simulink model "StereoImageRectificationHDL2020a"  (R2020a)
settings: Solver=FixedStepDiscrete  StartTime=0.0  StopTime=totalPixels*totalLines  FixedStep=1  RelTol=1e-3
InitFcn:
  | load('stereoParams.mat');
  | img = imread(get_param('StereoImageRectificationHDL2020a/LeftInputImage','FileName'));
  | dimOut=size(img);
  | [imgRowSize, imgColSize] = size(img);
  | run('ComputeRectificationParams.m');
values from neighbouring files (symbols this model uses):
  displacement = maxDev+firstRow    [ComputeRectificationParams.m]
  distCoeffsL = [this.CameraParameters1.RadialDistortion, this.CameraParameters1.TangentialDistortion]    [ComputeRectificationParams.m]
  distCoeffsR = [this.CameraParameters2.RadialDistortion, this.CameraParameters2.TangentialDistortion]    [ComputeRectificationParams.m]
  offset = displacement+50    [ComputeRectificationParams.m]
  recleftfx = 1/intrinsicL(1,1)    [ComputeRectificationParams.m]
  recleftfy = 1/intrinsicL(2,2)    [ComputeRectificationParams.m]
  recrightfx = 1/intrinsicR(1,1)    [ComputeRectificationParams.m]
  recrightfy = 1/intrinsicR(2,2)    [ComputeRectificationParams.m]
  totalLines = R + 100    (= 580)    [setup.m]
  totalPixels = C + frontPorch    (= 802)    [setup.m]
undefined symbols (not defined in the file or in its folder): gray, imgColSize, imgRowSize, intrinsicL, intrinsicR, leftH, rightH, XBounds, YBounds
libraries: simulink x62, hdlsllib x30, visionhdlio x4, visionsources x2, visionhdlutilities x1
(part 2 of 3)

== system StereoImageRectificationHDL2020a/HDLStereoImageRectification/RightUndistortion/Normalization ==
  yCoordinate : Inport
  xCoordinate : Inport  Port=2
  Add : Sum  Inputs=+-
  Add1 : Sum  Inputs=+-
  Constant : Constant  Value=intrinsic(2,3)  OutDataTypeStr=fixdt(1,ceil(log2(intrinsic(2,3)))+24,23)  SampleTime=-1
  Constant1 : Constant  Value=intrinsic(1,3)  OutDataTypeStr=fixdt(1,ceil(log2(intrinsic(1,3)))+24,23)  SampleTime=-1
  Constant2 : Constant  Value=recfy  OutDataTypeStr=Inherit: Inherit via back propagation  SampleTime=-1
  Constant3 : Constant  Value=recfx  OutDataTypeStr=Inherit: Inherit via back propagation  SampleTime=-1
  Delay{1..3,8} (4 alike) : Delay
  Delay30 : Delay  DelayLength=1
  Delay31 : Delay  DelayLength=1
  Product13 : Product  OutDataTypeStr=Inherit: Same as first input
  Product14 : Product  OutDataTypeStr=Inherit: Same as first input
  yNorm : Outport
  xNorm : Outport  Port=2
  wires:
  Delay2/1 -> xNorm/1
  Delay1/1 -> yNorm/1
  xCoordinate/1 -> Delay31/1
  Product14/1 -> Delay2/1  "xNorm"
  Add/1 -> Delay8/1
  Product13/1 -> Delay1/1  "yNorm"
  Delay30/1 -> Add/1
  Delay31/1 -> Add1/1
  Delay8/1 -> Product13/1
  yCoordinate/1 -> Delay30/1
  Constant2/1 -> Product13/2
  Constant3/1 -> Product14/2
  Constant/1 -> Add/2
  Add1/1 -> Delay3/1
  Delay3/1 -> Product14/1
  Constant1/1 -> Add1/2

== system StereoImageRectificationHDL2020a/HDLStereoImageRectification/RightUndistortion/ParameterCalculation ==
  yNorm : Inport
  xNorm : Inport  Port=2
  Add2 : Sum
  Delay{1..4,6..7,9} (7 alike) : Delay
  Product{,10..12} (4 alike) : Product  OutDataTypeStr=Inherit: Inherit via back propagation
  r4 : Outport
  r2 : Outport  Port=2
  xyProduct : Outport  Port=3
  xNorm2 : Outport  Port=4
  yNorm2 : Outport  Port=5
  wires:
  Delay4/1 -> xNorm2/1
  Delay3/1 -> yNorm2/1
  Delay2/1 -> xyProduct/1
  Delay1/1 -> Delay2/1
  xNorm/1 -> Product/2, Product11/1, Product11/2
  Product/1 -> Delay1/1  "xyProduct"
  yNorm/1 -> Product/1, Product10/2, Product10/1
  Add2/1 -> Delay9/1  "r2"
  Delay6/1 -> Delay3/1, Add2/1
  Delay7/1 -> Add2/2, Delay4/1
  Delay9/1 -> Product12/2, r2/1, Product12/1
  Product12/1 -> r4/1  "r4"
  Product11/1 -> Delay7/1  "xNorm2"
  Product10/1 -> Delay6/1  "yNorm2"

== system StereoImageRectificationHDL2020a/HDLStereoImageRectification/RightUndistortion/RadialDistortion ==
  r4 : Inport
  r2 : Inport  Port=2
  Add3 : Sum
  Delay{10..13,18} (5 alike) : Delay
  Product1 : Product  OutDataTypeStr=Inherit: Same as first input
  Product2 : Product  OutDataTypeStr=Inherit: Same as first input
  radial1 : Constant  Value=distCoeffs(1)  OutDataTypeStr=fixdt(1,17,16)  SampleTime=-1
  radial2 : Constant  Value=distCoeffs(2)  OutDataTypeStr=fixdt(1,17,16)  SampleTime=-1
  alpha : Outport
  wires:
  Delay10/1 -> Product1/1
  Delay12/1 -> Add3/1
  radial1/1 -> Product1/2
  Delay18/1 -> alpha/1
  Delay11/1 -> Product2/1
  Product2/1 -> Delay12/1
  r4/1 -> Delay11/1
  radial2/1 -> Product2/2
  Delay13/1 -> Add3/2
  Product1/1 -> Delay13/1
  Add3/1 -> Delay18/1  "alpha"
  r2/1 -> Delay10/1

== system StereoImageRectificationHDL2020a/HDLStereoImageRectification/RightUndistortion/dxTangential ==
  r2 : Inport
  xyProd : Inport  Port=2
  xNorm2 : Inport  Port=3
  Add : Sum
  Add1 : Sum
  Delay{,1..4,6..7} (7 alike) : Delay
  Delay5 : Delay  DelayLength=1
  Product : Product  OutDataTypeStr=Inherit: Same as first input
  Product2 : Product  OutDataTypeStr=Inherit: Same as first input  LockScale=on
  Shift Arithmetic : ArithShift  BitShiftNumber=1  BitShiftDirection=Left
  Shift Arithmetic1 : ArithShift  BitShiftNumber=1  BitShiftDirection=Left
  tangential1 : Constant  Value=distCoeffs(3)  OutDataTypeStr=fixdt(1,17,15)  SampleTime=-1
  tangential2 : Constant  Value=distCoeffs(4)  OutDataTypeStr=fixdt(1,17,15)  SampleTime=-1
  dxTan : Outport
  wires:
  Delay7/1 -> Delay3/1
  Delay6/1 -> Shift Arithmetic1/1
  tangential1/1 -> Product/2
  Shift Arithmetic1/1 -> Delay7/1
  Delay5/1 -> dxTan/1
  Add1/1 -> Delay5/1
  Delay4/1 -> Add1/2
  Product2/1 -> Delay4/1
  Delay3/1 -> Add1/1
  Product/1 -> Delay6/1
  tangential2/1 -> Product2/2
  Delay2/1 -> Product2/1
  Add/1 -> Delay2/1
  Delay1/1 -> Add/2
  r2/1 -> Delay1/1
  Delay/1 -> Add/1
  Shift Arithmetic/1 -> Delay/1
  xNorm2/1 -> Shift Arithmetic/1
  xyProd/1 -> Product/1

== system StereoImageRectificationHDL2020a/HDLStereoImageRectification/RightUndistortion/dyTangential ==
  r2 : Inport
  xyProd : Inport  Port=2
  yNorm2 : Inport  Port=3
  Add : Sum
  Add1 : Sum
  Delay{,1..4,6..7} (7 alike) : Delay
  Delay5 : Delay  DelayLength=1
  Product : Product  OutDataTypeStr=Inherit: Same as first input
  Product2 : Product  OutDataTypeStr=Inherit: Same as first input
  Shift Arithmetic : ArithShift  BitShiftNumber=1  BitShiftDirection=Left
  Shift Arithmetic1 : ArithShift  BitShiftNumber=1  BitShiftDirection=Left
  tangential1 : Constant  Value=distCoeffs(3)  OutDataTypeStr=fixdt(1,17,15)  SampleTime=-1
  tangential2 : Constant  Value=distCoeffs(4)  OutDataTypeStr=fixdt(1,17,15)  SampleTime=-1
  dyTan : Outport
  wires:
  Delay7/1 -> Delay3/1
  Delay6/1 -> Shift Arithmetic1/1
  Product/1 -> Delay6/1
  Shift Arithmetic1/1 -> Delay7/1
  Delay5/1 -> dyTan/1
  Add1/1 -> Delay5/1
  Delay4/1 -> Add1/2
  Product2/1 -> Delay4/1
  Delay3/1 -> Add1/1
  tangential1/1 -> Product2/2
  Delay2/1 -> Product2/1
  Add/1 -> Delay2/1
  Delay1/1 -> Add/2
  r2/1 -> Delay1/1
  Delay/1 -> Add/1
  Shift Arithmetic/1 -> Delay/1
  yNorm2/1 -> Shift Arithmetic/1
  tangential2/1 -> Product/2
  xyProd/1 -> Product/1

== system StereoImageRectificationHDL2020a/HDLStereoImageRectification/LeftInterpolation/AddressGeneration/AddressCalculation ==
  col : Inport
  row : Inport  Port=2
  Add4 : Sum  OutDataTypeStr=Inherit: Same as first input
  CappingAddress : Subsystem
  Constant2 : Constant  OutDataTypeStr=Inherit: Inherit via back propagation  SampleTime=-1
  Delay{,1..3} (4 alike) : Delay  DelayLength=3
  IndexChangeForMemoryAccess : MATLAB Function  TreatAsAtomicUnit=on
  Pix1Add : Subsystem
  Pix2Add : Subsystem
  Pix3Add : Subsystem
  Pix4Add : Subsystem
  Vector Concatenate : Concatenate  NumInputs=4
  Vector Concatenate1 : Concatenate  NumInputs=4
  leftAdd : Outport
  leftIndex : Outport  Port=2
  wires:
  Constant2/1 -> Add4/2
  IndexChangeForMemoryAccess/1(Add_Re) -> leftAdd/1
  Vector Concatenate/1 -> IndexChangeForMemoryAccess/1(add)
  Vector Concatenate1/1 -> IndexChangeForMemoryAccess/2(index)
  row/1 -> CappingAddress/1(row)
  col/1 -> CappingAddress/2(col)
  CappingAddress/1(r) -> Add4/1, Pix1Add/1(row)
  CappingAddress/2(c) -> Pix3Add/2(col), Pix1Add/2(col)
  IndexChangeForMemoryAccess/2(Index_Re) -> leftIndex/1
  Pix1Add/1(A1) -> Pix2Add/1(A1), Delay/1
  Pix1Add/2(index) -> Pix2Add/2(Index), Delay2/1
  Add4/1 -> Pix3Add/1(row)
  Pix3Add/1(A3) -> Pix4Add/1(A3), Delay1/1
  Pix3Add/2(index) -> Pix4Add/2(Index), Delay3/1
  Pix2Add/1(A2) -> Vector Concatenate/2
  Pix2Add/2(index) -> Vector Concatenate1/2
  Pix4Add/2(index) -> Vector Concatenate1/4
  Pix4Add/1(A4) -> Vector Concatenate/4
  Delay/1 -> Vector Concatenate/1
  Delay1/1 -> Vector Concatenate/3
  Delay2/1 -> Vector Concatenate1/1
  Delay3/1 -> Vector Concatenate1/3

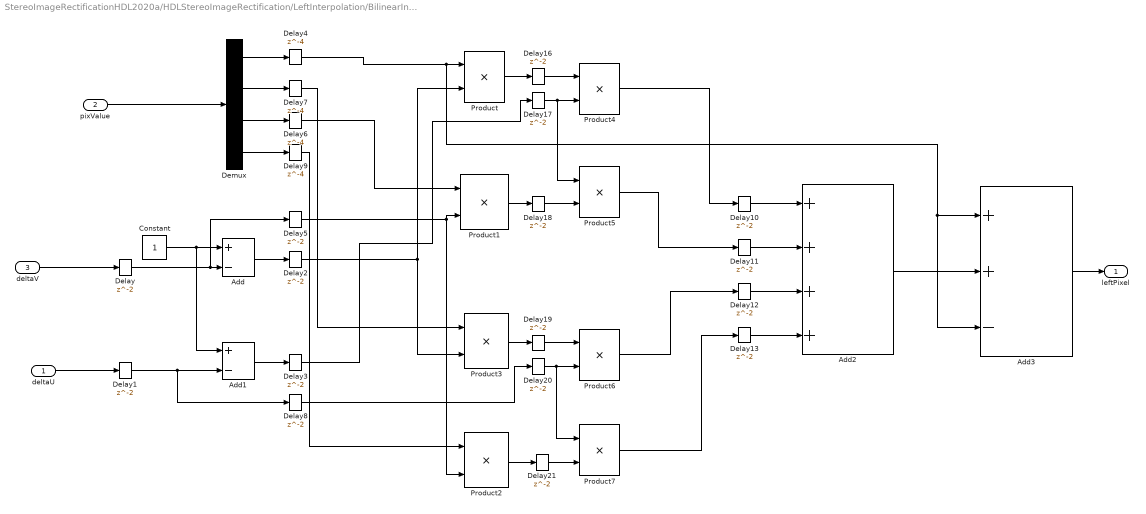
== system StereoImageRectificationHDL2020a/HDLStereoImageRectification/LeftInterpolation/BilinearInterpolation/BilinearInterpolationEquation ==
  deltaU : Inport
  pixValue : Inport  Port=2
  deltaV : Inport  Port=3
  Add : Sum  Inputs=+-  OutDataTypeStr=Inherit: Inherit via back propagation
  Add1 : Sum  Inputs=+-  OutDataTypeStr=Inherit: Inherit via back propagation
  Add2 : Sum  Inputs=++++  OutDataTypeStr=Inherit: Inherit via back propagation  RndMeth=Nearest
  Add3 : Sum  Inputs=++-  RndMeth=Nearest  OutDataTypeStr=Inherit: Same as first input
  Constant : Constant  OutDataTypeStr=Inherit: Inherit via back propagation  SampleTime=-1
  Delay{,1..3,5,8,10..13,16..21} (16 alike) : Delay
  Delay{4,6..7,9} (4 alike) : Delay  DelayLength=4
  Demux : Demux
  Product{,1..3} (4 alike) : Product  LockScale=on
  Product{4..7} (4 alike) : Product  OutDataTypeStr=Inherit: Inherit via back propagation  LockScale=on
  leftPixel : Outport
  wires:
  pixValue/1 -> Demux/1
  deltaV/1 -> Delay/1
  deltaU/1 -> Delay1/1
  Constant/1 -> Add1/1, Add/1
  Add/1 -> Delay2/1
  Add1/1 -> Delay3/1
  Delay2/1 -> Product3/2, Product/2
  Delay3/1 -> Delay17/1
  Demux/1 -> Delay4/1
  Delay4/1 -> Add3/3, Add3/1, Product/1
  Demux/3 -> Delay6/1
  Delay5/1 -> Product2/2, Product1/2
  Delay6/1 -> Product1/1
  Demux/2 -> Delay7/1
  Delay7/1 -> Product3/1
  Delay1/1 -> Add1/2, Delay8/1
  Delay8/1 -> Delay20/1
  Demux/4 -> Delay9/1
  Delay9/1 -> Product2/1
  Product/1 -> Delay16/1
  Product1/1 -> Delay18/1
  Product3/1 -> Delay19/1
  Product2/1 -> Delay21/1
  Delay10/1 -> Add2/1
  Delay11/1 -> Add2/2
  Delay12/1 -> Add2/3
  Delay13/1 -> Add2/4
  Delay/1 -> Delay5/1, Add/2
  Delay16/1 -> Product4/1
  Delay17/1 -> Product5/1, Product4/2
  Product4/1 -> Delay10/1
  Delay18/1 -> Product5/2
  Product5/1 -> Delay11/1
  Delay19/1 -> Product6/1
  Delay20/1 -> Product7/1, Product6/2
  Product6/1 -> Delay12/1
  Delay21/1 -> Product7/2
  Product7/1 -> Delay13/1
  Add3/1 -> leftPixel/1
  Add2/1 -> Add3/2

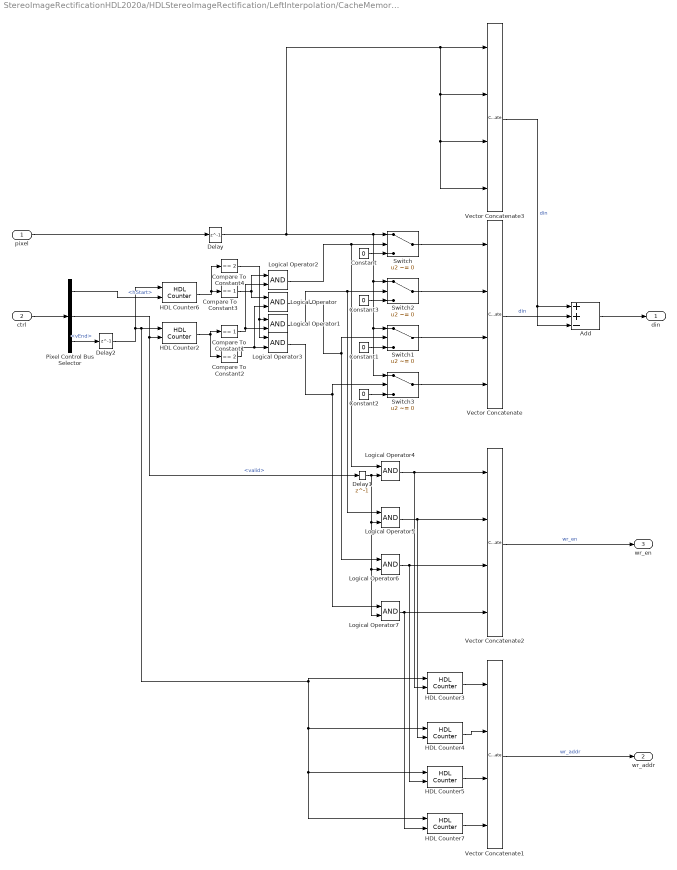
== system StereoImageRectificationHDL2020a/HDLStereoImageRectification/LeftInterpolation/CacheMemory/WriteControl ==
  pixel : Inport
  ctrl : Inport  Port=2
  Add : Sum  Inputs=++-  OutDataTypeStr=Inherit: Same as first input
  Compare To Constant1 : simulink/Logic and Bit Operations/Compare To Constant  relop===  const=1  OutDataTypeStr=boolean
  Compare To Constant2 : simulink/Logic and Bit Operations/Compare To Constant  relop===  const=2  OutDataTypeStr=boolean
  Compare To Constant3 : simulink/Logic and Bit Operations/Compare To Constant  relop===  const=1  OutDataTypeStr=boolean
  Compare To Constant4 : simulink/Logic and Bit Operations/Compare To Constant  relop===  const=2  OutDataTypeStr=boolean
  Constant{,1..3} (4 alike) : Constant  Value=0  OutDataTypeStr=Inherit: Inherit via back propagation  SampleTime=-1
  Delay : Delay  DelayLength=1
  Delay1 : Delay  DelayLength=1
  Delay2 : Delay  DelayLength=1
  HDL Counter2 : hdlsllib/Sources/HDL Counter  CountType=Count limited  CountInit=2  CountStep=1  CountMax=2  CountFromType=Specify  CountFrom=1  CountResetPort=on  CountLoadPort=off  CountEnbPort=on  CountDirPort=off  CountDataType=Unsigned  CountWordLen=3  CountFracLen=0  CountSampTime=1
  HDL Counter{3..5,7} (4 alike) : hdlsllib/Sources/HDL Counter  CountType=Count limited  CountInit=1  CountStep=1  CountMax=offset*dimOut(2)/4  CountFromType=Specify  CountFrom=1  CountResetPort=on  CountLoadPort=off  CountEnbPort=on  CountDirPort=off  CountDataType=Unsigned  CountWordLen=ceil(log2(offset*dimOut(2)/4))  CountFracLen=0  CountSampTime=1
  HDL Counter6 : hdlsllib/Sources/HDL Counter  CountType=Count limited  CountInit=2  CountStep=1  CountMax=2  CountFromType=Specify  CountFrom=1  CountResetPort=on  CountLoadPort=off  CountEnbPort=on  CountDirPort=off  CountDataType=Unsigned  CountWordLen=3  CountFracLen=0  CountSampTime=1
  Logical Operator{,1..7} (8 alike) : Logic  AllPortsSameDT=off  OutDataTypeStr=boolean
  Pixel Control Bus Selector : BusSelector  OutputSignals=hStart,valid,vEnd
  Switch{,1..3} (4 alike) : Switch  Criteria=u2 ~= 0
  Vector Concatenate{,1..3} (4 alike) : Concatenate  NumInputs=4
  din : Outport  VectorParamsAs1DForOutWhenUnconnected=off
  wr_addr : Outport  Port=2  VectorParamsAs1DForOutWhenUnconnected=off
  wr_en : Outport  Port=3  VectorParamsAs1DForOutWhenUnconnected=off
  wires:
  Vector Concatenate/1 -> Add/2  "din"
  ctrl/1 -> Pixel Control Bus Selector/1
  Constant/1 -> Switch/3
  Switch1/1 -> Vector Concatenate/3
  Switch/1 -> Vector Concatenate/1
  Constant1/1 -> Switch1/3
  pixel/1 -> Delay/1
  Pixel Control Bus Selector/2 -> Delay1/1, HDL Counter2/2  "<valid>"
  Vector Concatenate1/1 -> wr_addr/1  "wr_addr"
  Vector Concatenate2/1 -> wr_en/1  "wr_en"
  Pixel Control Bus Selector/1 -> HDL Counter6/2  "<hStart>"
  HDL Counter6/1 -> Compare To Constant4/1, Compare To Constant3/1
  HDL Counter2/1 -> Compare To Constant1/1, Compare To Constant2/1
  Switch2/1 -> Vector Concatenate/2
  Switch3/1 -> Vector Concatenate/4
  Delay/1 -> Vector Concatenate3/4, Vector Concatenate3/3, Vector Concatenate3/2, Vector Concatenate3/1, Switch2/1, Switch3/1, Switch1/1, Switch/1
  Constant2/1 -> Switch3/3
  Constant3/1 -> Switch2/3
  Compare To Constant3/1 -> Logical Operator/1, Logical Operator2/1
  Compare To Constant1/1 -> Logical Operator1/2, Logical Operator2/2
  Logical Operator2/1 -> Logical Operator4/1, Switch/2
  Compare To Constant2/1 -> Logical Operator3/2, Logical Operator/2
  Logical Operator/1 -> Logical Operator6/1, Switch1/2
  Compare To Constant4/1 -> Logical Operator3/1, Logical Operator1/1
  Logical Operator1/1 -> Logical Operator5/1, Switch2/2
  Logical Operator3/1 -> Logical Operator7/1, Switch3/2
  Delay1/1 -> Logical Operator7/2, Logical Operator6/2, Logical Operator5/2, Logical Operator4/2
  Logical Operator4/1 -> Vector Concatenate2/1, HDL Counter3/2
  Logical Operator5/1 -> HDL Counter4/2, Vector Concatenate2/2
  Logical Operator6/1 -> HDL Counter5/2, Vector Concatenate2/3
  Logical Operator7/1 -> HDL Counter7/2, Vector Concatenate2/4
  HDL Counter3/1 -> Vector Concatenate1/1
  HDL Counter4/1 -> Vector Concatenate1/2
  HDL Counter5/1 -> Vector Concatenate1/3
  HDL Counter7/1 -> Vector Concatenate1/4
  Add/1 -> din/1
  Pixel Control Bus Selector/3 -> Delay2/1  "<vEnd>"
  Delay2/1 -> HDL Counter6/1, HDL Counter4/1, HDL Counter7/1, HDL Counter5/1, HDL Counter3/1, HDL Counter2/1
  Vector Concatenate3/1 -> Add/3, Add/1  "din"

== system StereoImageRectificationHDL2020a/HDLStereoImageRectification/RightInterpolation/AddressGeneration/AddressCalculation ==
  col : Inport
  row : Inport  Port=2
  Add4 : Sum  OutDataTypeStr=Inherit: Same as first input
  CappingAddress : Subsystem
  Constant2 : Constant  OutDataTypeStr=Inherit: Inherit via back propagation  SampleTime=-1
  Delay{,1..3} (4 alike) : Delay  DelayLength=3
  IndexChangeForMemoryAccess : MATLAB Function  TreatAsAtomicUnit=on
  Pix1Add : Subsystem
  Pix2Add : Subsystem
  Pix3Add : Subsystem
  Pix4Add : Subsystem
  Vector Concatenate : Concatenate  NumInputs=4
  Vector Concatenate1 : Concatenate  NumInputs=4
  leftAdd : Outport
  leftIndex : Outport  Port=2
  wires:
  Constant2/1 -> Add4/2
  IndexChangeForMemoryAccess/1(Add_Re) -> leftAdd/1
  Vector Concatenate/1 -> IndexChangeForMemoryAccess/1(add)
  Vector Concatenate1/1 -> IndexChangeForMemoryAccess/2(index)
  row/1 -> CappingAddress/1(row)
  col/1 -> CappingAddress/2(col)
  CappingAddress/1(r) -> Add4/1, Pix1Add/1(row)
  CappingAddress/2(c) -> Pix3Add/2(col), Pix1Add/2(col)
  IndexChangeForMemoryAccess/2(Index_Re) -> leftIndex/1
  Pix1Add/1(A1) -> Pix2Add/1(A1), Delay/1
  Pix1Add/2(index) -> Pix2Add/2(Index), Delay2/1
  Add4/1 -> Pix3Add/1(row)
  Pix3Add/1(A3) -> Pix4Add/1(A3), Delay1/1
  Pix3Add/2(index) -> Pix4Add/2(Index), Delay3/1
  Pix2Add/1(A2) -> Vector Concatenate/2
  Pix2Add/2(index) -> Vector Concatenate1/2
  Pix4Add/2(index) -> Vector Concatenate1/4
  Pix4Add/1(A4) -> Vector Concatenate/4
  Delay/1 -> Vector Concatenate/1
  Delay1/1 -> Vector Concatenate/3
  Delay2/1 -> Vector Concatenate1/1
  Delay3/1 -> Vector Concatenate1/3

== system StereoImageRectificationHDL2020a/HDLStereoImageRectification/RightInterpolation/BilinearInterpolation/BilinearInterpolationEquation ==
  deltaU : Inport
  pixValue : Inport  Port=2
  deltaV : Inport  Port=3
  Add : Sum  Inputs=+-  OutDataTypeStr=Inherit: Inherit via back propagation
  Add1 : Sum  Inputs=+-  OutDataTypeStr=Inherit: Inherit via back propagation
  Add2 : Sum  Inputs=++++  OutDataTypeStr=Inherit: Inherit via back propagation  RndMeth=Nearest
  Add3 : Sum  Inputs=++-  RndMeth=Nearest  OutDataTypeStr=Inherit: Same as first input
  Constant : Constant  OutDataTypeStr=Inherit: Inherit via back propagation  SampleTime=-1
  Delay{,1..3,5,8,10..13,16..21} (16 alike) : Delay
  Delay{4,6..7,9} (4 alike) : Delay  DelayLength=4
  Demux : Demux
  Product{,1..3} (4 alike) : Product  LockScale=on
  Product{4..7} (4 alike) : Product  OutDataTypeStr=Inherit: Inherit via back propagation  LockScale=on
  leftPixel : Outport
  wires:
  pixValue/1 -> Demux/1
  deltaV/1 -> Delay/1
  deltaU/1 -> Delay1/1
  Constant/1 -> Add1/1, Add/1
  Add/1 -> Delay2/1
  Add1/1 -> Delay3/1
  Delay2/1 -> Product3/2, Product/2
  Delay3/1 -> Delay17/1
  Demux/1 -> Delay4/1
  Delay4/1 -> Add3/3, Add3/1, Product/1
  Demux/3 -> Delay6/1
  Delay5/1 -> Product2/2, Product1/2
  Delay6/1 -> Product1/1
  Demux/2 -> Delay7/1
  Delay7/1 -> Product3/1
  Delay1/1 -> Add1/2, Delay8/1
  Delay8/1 -> Delay20/1
  Demux/4 -> Delay9/1
  Delay9/1 -> Product2/1
  Product/1 -> Delay16/1
  Product1/1 -> Delay18/1
  Product3/1 -> Delay19/1
  Product2/1 -> Delay21/1
  Delay10/1 -> Add2/1
  Delay11/1 -> Add2/2
  Delay12/1 -> Add2/3
  Delay13/1 -> Add2/4
  Delay/1 -> Delay5/1, Add/2
  Delay16/1 -> Product4/1
  Delay17/1 -> Product5/1, Product4/2
  Product4/1 -> Delay10/1
  Delay18/1 -> Product5/2
  Product5/1 -> Delay11/1
  Delay19/1 -> Product6/1
  Delay20/1 -> Product7/1, Product6/2
  Product6/1 -> Delay12/1
  Delay21/1 -> Product7/2
  Product7/1 -> Delay13/1
  Add3/1 -> leftPixel/1
  Add2/1 -> Add3/2

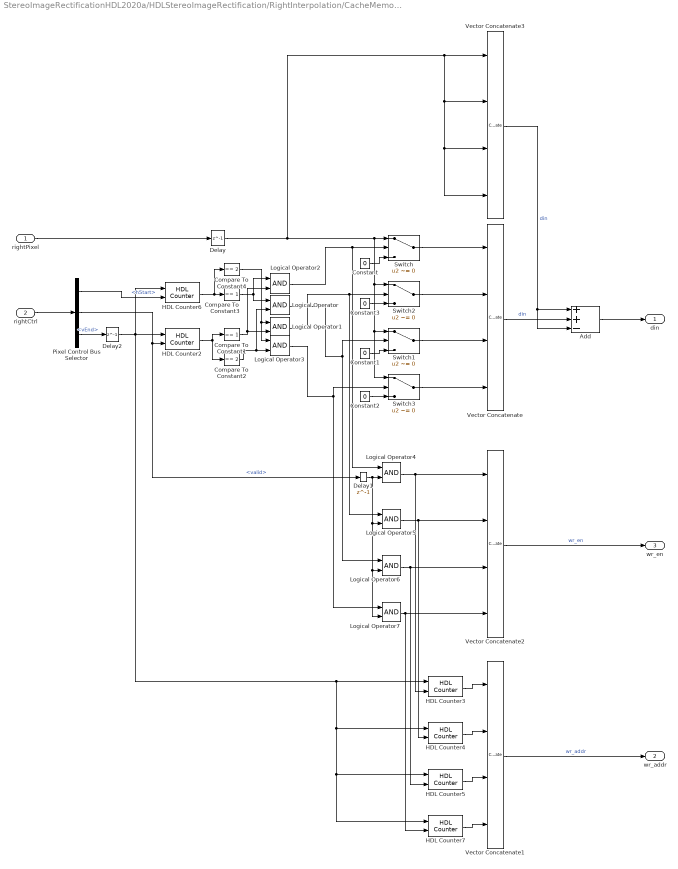
== system StereoImageRectificationHDL2020a/HDLStereoImageRectification/RightInterpolation/CacheMemory/RightWriteControl ==
  rightPixel : Inport
  rightCtrl : Inport  Port=2
  Add : Sum  Inputs=++-  OutDataTypeStr=Inherit: Same as first input
  Compare To Constant1 : simulink/Logic and Bit Operations/Compare To Constant  relop===  const=1  OutDataTypeStr=boolean
  Compare To Constant2 : simulink/Logic and Bit Operations/Compare To Constant  relop===  const=2  OutDataTypeStr=boolean
  Compare To Constant3 : simulink/Logic and Bit Operations/Compare To Constant  relop===  const=1  OutDataTypeStr=boolean
  Compare To Constant4 : simulink/Logic and Bit Operations/Compare To Constant  relop===  const=2  OutDataTypeStr=boolean
  Constant{,1..3} (4 alike) : Constant  Value=0  OutDataTypeStr=Inherit: Inherit via back propagation  SampleTime=-1
  Delay : Delay  DelayLength=1
  Delay1 : Delay  DelayLength=1
  Delay2 : Delay  DelayLength=1
  HDL Counter2 : hdlsllib/Sources/HDL Counter  CountType=Count limited  CountInit=2  CountStep=1  CountMax=2  CountFromType=Specify  CountFrom=1  CountResetPort=on  CountLoadPort=off  CountEnbPort=on  CountDirPort=off  CountDataType=Unsigned  CountWordLen=3  CountFracLen=0  CountSampTime=1
  HDL Counter{3..5,7} (4 alike) : hdlsllib/Sources/HDL Counter  CountType=Count limited  CountInit=1  CountStep=1  CountMax=offset*dimOut(2)/4  CountFromType=Specify  CountFrom=1  CountResetPort=on  CountLoadPort=off  CountEnbPort=on  CountDirPort=off  CountDataType=Unsigned  CountWordLen=ceil(log2(offset*dimOut(2)/4))  CountFracLen=0  CountSampTime=1
  HDL Counter6 : hdlsllib/Sources/HDL Counter  CountType=Count limited  CountInit=2  CountStep=1  CountMax=2  CountFromType=Specify  CountFrom=1  CountResetPort=on  CountLoadPort=off  CountEnbPort=on  CountDirPort=off  CountDataType=Unsigned  CountWordLen=3  CountFracLen=0  CountSampTime=1
  Logical Operator{,1..7} (8 alike) : Logic  AllPortsSameDT=off  OutDataTypeStr=boolean
  Pixel Control Bus Selector : BusSelector  OutputSignals=hStart,valid,vEnd
  Switch{,1..3} (4 alike) : Switch  Criteria=u2 ~= 0
  Vector Concatenate{,1..3} (4 alike) : Concatenate  NumInputs=4
  din : Outport  VectorParamsAs1DForOutWhenUnconnected=off
  wr_addr : Outport  Port=2  VectorParamsAs1DForOutWhenUnconnected=off
  wr_en : Outport  Port=3  VectorParamsAs1DForOutWhenUnconnected=off
  wires:
  Add/1 -> din/1
  HDL Counter7/1 -> Vector Concatenate1/4
  HDL Counter5/1 -> Vector Concatenate1/3
  HDL Counter4/1 -> Vector Concatenate1/2
  HDL Counter3/1 -> Vector Concatenate1/1
  Logical Operator7/1 -> Vector Concatenate2/4, HDL Counter7/2
  Logical Operator6/1 -> Vector Concatenate2/3, HDL Counter5/2
  Logical Operator5/1 -> Vector Concatenate2/2, HDL Counter4/2
  Logical Operator4/1 -> HDL Counter3/2, Vector Concatenate2/1
  Delay1/1 -> Logical Operator4/2, Logical Operator5/2, Logical Operator6/2, Logical Operator7/2
  Logical Operator3/1 -> Switch3/2, Logical Operator7/1
  Logical Operator1/1 -> Switch2/2, Logical Operator5/1
  Compare To Constant4/1 -> Logical Operator1/1, Logical Operator3/1
  Logical Operator/1 -> Switch1/2, Logical Operator6/1
  Compare To Constant2/1 -> Logical Operator/2, Logical Operator3/2
  Logical Operator2/1 -> Switch/2, Logical Operator4/1
  Compare To Constant1/1 -> Logical Operator2/2, Logical Operator1/2
  Compare To Constant3/1 -> Logical Operator2/1, Logical Operator/1
  Constant3/1 -> Switch2/3
  Constant2/1 -> Switch3/3
  Delay/1 -> Vector Concatenate3/3, Vector Concatenate3/4, Vector Concatenate3/2, Vector Concatenate3/1, Switch/1, Switch3/1, Switch1/1, Switch2/1
  Switch3/1 -> Vector Concatenate/4
  Switch2/1 -> Vector Concatenate/2
  HDL Counter2/1 -> Compare To Constant1/1, Compare To Constant2/1
  HDL Counter6/1 -> Compare To Constant3/1, Compare To Constant4/1
  Pixel Control Bus Selector/1 -> HDL Counter6/2  "<hStart>"
  Vector Concatenate2/1 -> wr_en/1  "wr_en"
  Vector Concatenate1/1 -> wr_addr/1  "wr_addr"
  Pixel Control Bus Selector/2 -> HDL Counter2/2, Delay1/1  "<valid>"
  rightPixel/1 -> Delay/1
  Constant1/1 -> Switch1/3
  Switch/1 -> Vector Concatenate/1
  Switch1/1 -> Vector Concatenate/3
  Constant/1 -> Switch/3
  rightCtrl/1 -> Pixel Control Bus Selector/1
  Vector Concatenate/1 -> Add/2  "din"
  Pixel Control Bus Selector/3 -> Delay2/1  "<vEnd>"
  Delay2/1 -> HDL Counter5/1, HDL Counter7/1, HDL Counter4/1, HDL Counter3/1, HDL Counter6/1, HDL Counter2/1
  Vector Concatenate3/1 -> Add/3, Add/1  "din"

== system StereoImageRectificationHDL2020a/HDLStereoImageRectification/LeftInterpolation/AddressGeneration/AddressCalculation/CappingAddress ==
  row : Inport
  col : Inport  Port=2
  AND1 : Logic  IconShape=distinctive  AllPortsSameDT=off  OutDataTypeStr=boolean
  AND2 : Logic  IconShape=distinctive  AllPortsSameDT=off  OutDataTypeStr=boolean
  Compare To Constant3 : simulink/Logic and Bit Operations/Compare To Constant  relop=<=  const=1  OutDataTypeStr=boolean
  Compare To Constant4 : simulink/Logic and Bit Operations/Compare To Constant  relop=<=  const=dimOut(2)-1  OutDataTypeStr=boolean
  Compare To Constant5 : simulink/Logic and Bit Operations/Compare To Constant  relop=>  const=1  OutDataTypeStr=boolean
  Compare To Constant6 : simulink/Logic and Bit Operations/Compare To Constant  relop=<=  const=1  OutDataTypeStr=boolean
  Compare To Constant7 : simulink/Logic and Bit Operations/Compare To Constant  relop=<=  const=dimOut(1)-1  OutDataTypeStr=boolean
  Compare To Constant8 : simulink/Logic and Bit Operations/Compare To Constant  relop=>  const=1  OutDataTypeStr=boolean
  Constant1 : Constant  Value=dimOut(2)-1  OutDataTypeStr=Inherit: Inherit via back propagation  SampleTime=-1
  Constant2 : Constant  Value=dimOut(1)-1  OutDataTypeStr=Inherit: Inherit via back propagation  SampleTime=-1
  Constant3 : Constant  OutDataTypeStr=Inherit: Inherit via back propagation  SampleTime=-1
  Constant4 : Constant  OutDataTypeStr=Inherit: Inherit via back propagation  SampleTime=-1
  Delay{,1..17} (18 alike) : Delay  DelayLength=1
  Switch{2..5} (4 alike) : Switch  Criteria=u2 ~= 0  OutDataTypeStr=Inherit: Inherit via back propagation
  r : Outport
  c : Outport  Port=2
  wires:
  col/1 -> Compare To Constant5/1, Compare To Constant4/1, Delay3/1, Delay6/1
  Compare To Constant5/1 -> Delay1/1
  Switch2/1 -> Delay5/1
  Constant3/1 -> Switch3/1
  Compare To Constant4/1 -> Delay/1
  AND1/1 -> Delay2/1
  Constant1/1 -> Switch2/3
  Compare To Constant3/1 -> Delay8/1
  Delay/1 -> AND1/1
  Delay1/1 -> AND1/2
  Delay2/1 -> Switch2/2
  Delay3/1 -> Delay4/1
  Delay4/1 -> Switch2/1
  Delay5/1 -> Switch3/3
  Delay6/1 -> Delay7/1
  Delay7/1 -> Compare To Constant3/1
  Delay8/1 -> Switch3/2
  Delay17/1 -> Switch5/2
  Delay10/1 -> AND2/2
  Delay14/1 -> Switch5/3
  Delay15/1 -> Delay16/1
  Delay12/1 -> Delay13/1
  Delay13/1 -> Switch4/1
  Delay11/1 -> Switch4/2
  Delay16/1 -> Compare To Constant6/1
  Switch4/1 -> Delay14/1
  row/1 -> Delay15/1, Compare To Constant8/1, Compare To Constant7/1, Delay12/1
  Compare To Constant8/1 -> Delay10/1
  Constant2/1 -> Switch4/3
  AND2/1 -> Delay11/1
  Compare To Constant6/1 -> Delay17/1
  Constant4/1 -> Switch5/1
  Compare To Constant7/1 -> Delay9/1
  Delay9/1 -> AND2/1
  Switch3/1 -> c/1
  Switch5/1 -> r/1

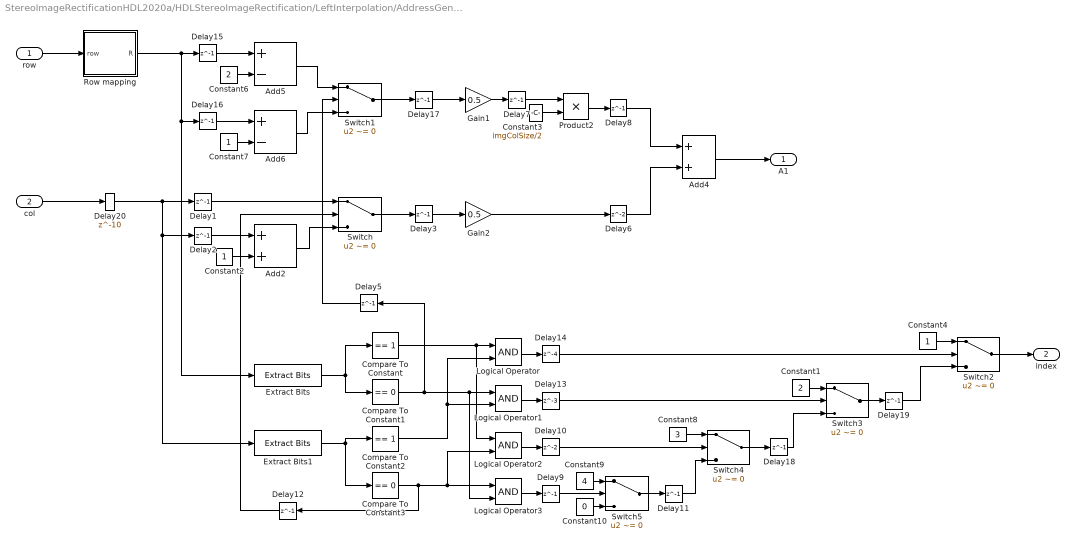
== system StereoImageRectificationHDL2020a/HDLStereoImageRectification/LeftInterpolation/AddressGeneration/AddressCalculation/Pix1Add ==
  row : Inport
  col : Inport  Port=2
  Add2 : Sum  OutDataTypeStr=Inherit: Same as first input
  Add4 : Sum  OutDataTypeStr=Inherit: Same as first input
  Add5 : Sum  Inputs=+-  OutDataTypeStr=Inherit: Same as first input
  Add6 : Sum  Inputs=+-  OutDataTypeStr=Inherit: Same as first input
  Compare To Constant : simulink/Logic and Bit Operations/Compare To Constant  relop===  const=1  OutDataTypeStr=boolean
  Compare To Constant1 : simulink/Logic and Bit Operations/Compare To Constant  relop===  const=0  OutDataTypeStr=boolean
  Compare To Constant2 : simulink/Logic and Bit Operations/Compare To Constant  relop===  const=1  OutDataTypeStr=boolean
  Compare To Constant3 : simulink/Logic and Bit Operations/Compare To Constant  relop===  const=0  OutDataTypeStr=boolean
  Constant1 : Constant  Value=2  OutDataTypeStr=uint8  SampleTime=-1
  Constant10 : Constant  Value=0  OutDataTypeStr=uint8  SampleTime=-1
  Constant2 : Constant  OutDataTypeStr=Inherit: Inherit via back propagation  SampleTime=-1
  Constant3 : Constant  Value=imgColSize/2  OutDataTypeStr=uint32  SampleTime=-1
  Constant4 : Constant  OutDataTypeStr=uint8  SampleTime=-1
  Constant6 : Constant  Value=2  OutDataTypeStr=Inherit: Inherit via back propagation  SampleTime=-1
  Constant7 : Constant  OutDataTypeStr=Inherit: Inherit via back propagation  SampleTime=-1
  Constant8 : Constant  Value=3  OutDataTypeStr=uint8  SampleTime=-1
  Constant9 : Constant  Value=4  OutDataTypeStr=uint8  SampleTime=-1
  Delay{1..3,5,7..9,11..12,15..19} (14 alike) : Delay  DelayLength=1
  Delay10 : Delay
  Delay13 : Delay  DelayLength=3
  Delay14 : Delay  DelayLength=4
  Delay20 : Delay  DelayLength=10
  Delay6 : Delay
  Extract Bits : simulink/Logic and Bit Operations/Extract Bits  bitsToExtract=Range ending with least significant bit  numBits=1  bitIdxRange=[0 7]  outScalingMode=Preserve fixed-point scaling
  Extract Bits1 : simulink/Logic and Bit Operations/Extract Bits  bitsToExtract=Range ending with least significant bit  numBits=1  bitIdxRange=[0 7]  outScalingMode=Preserve fixed-point scaling
  Gain1 : Gain  Gain=0.5  OutDataTypeStr=Inherit: Inherit via back propagation
  Gain2 : Gain  Gain=0.5  OutDataTypeStr=Inherit: Inherit via back propagation
  Logical Operator{,1..3} (4 alike) : Logic  AllPortsSameDT=off  OutDataTypeStr=boolean
  Product2 : Product  OutDataTypeStr=Inherit: Inherit via back propagation
  Row mapping : Subsystem
  Switch{,1..5} (6 alike) : Switch  Criteria=u2 ~= 0
  A1 : Outport
  index : Outport  Port=2
  wires:
  col/1 -> Delay20/1
  Delay12/1 -> Switch/2
  Compare To Constant3/1 -> Delay12/1, Logical Operator2/2, Logical Operator3/1
  Switch2/1 -> index/1
  Logical Operator3/1 -> Delay9/1
  Logical Operator2/1 -> Delay10/1
  Logical Operator1/1 -> Delay13/1
  Logical Operator/1 -> Delay14/1
  Compare To Constant1/1 -> Logical Operator1/1, Logical Operator3/2, Delay5/1
  Compare To Constant2/1 -> Logical Operator/2, Logical Operator1/2
  Compare To Constant/1 -> Logical Operator/1, Logical Operator2/1
  Extract Bits1/1 -> Compare To Constant3/1, Compare To Constant2/1
  Extract Bits/1 -> Compare To Constant/1, Compare To Constant1/1
  Add4/1 -> A1/1
  Delay6/1 -> Add4/2
  Delay8/1 -> Add4/1
  Product2/1 -> Delay8/1
  Delay7/1 -> Product2/1
  Constant3/1 -> Product2/2
  Gain1/1 -> Delay7/1
  Constant6/1 -> Add5/2
  Delay15/1 -> Add5/1
  Delay16/1 -> Add6/1
  Constant7/1 -> Add6/2
  row/1 -> Row mapping/1(row)
  Add5/1 -> Switch1/1
  Add6/1 -> Switch1/3
  Switch1/1 -> Delay17/1
  Delay17/1 -> Gain1/1
  Delay5/1 -> Switch1/2
  Add2/1 -> Switch/3
  Delay1/1 -> Switch/1
  Constant2/1 -> Add2/2
  Delay2/1 -> Add2/1
  Delay3/1 -> Gain2/1
  Switch/1 -> Delay3/1
  Gain2/1 -> Delay6/1
  Constant1/1 -> Switch3/1
  Constant4/1 -> Switch2/1
  Switch3/1 -> Delay19/1
  Switch4/1 -> Delay18/1
  Constant8/1 -> Switch4/1
  Constant9/1 -> Switch5/1
  Switch5/1 -> Delay11/1
  Constant10/1 -> Switch5/3
  Delay9/1 -> Switch5/2
  Delay10/1 -> Switch4/2
  Delay13/1 -> Switch3/2
  Delay14/1 -> Switch2/2
  Delay11/1 -> Switch4/3
  Delay18/1 -> Switch3/3
  Delay19/1 -> Switch2/3
  Row mapping/1(R) -> Extract Bits/1, Delay16/1, Delay15/1
  Delay20/1 -> Extract Bits1/1, Delay2/1, Delay1/1

== system StereoImageRectificationHDL2020a/HDLStereoImageRectification/LeftInterpolation/AddressGeneration/AddressCalculation/Pix2Add ==
  A1 : Inport
  Index : Inport  Port=2
  Add : Sum  OutDataTypeStr=Inherit: Inherit via back propagation
  Add2 : Sum  OutDataTypeStr=Inherit: Inherit via back propagation
  Add3 : Sum  Inputs=+-  OutDataTypeStr=Inherit: Inherit via back propagation
  Compare To Constant : simulink/Logic and Bit Operations/Compare To Constant  relop===  const=1  OutDataTypeStr=boolean
  Compare To Constant1 : simulink/Logic and Bit Operations/Compare To Constant  relop===  const=2  OutDataTypeStr=boolean
  Constant : Constant  OutDataTypeStr=Inherit: Inherit via back propagation  SampleTime=-1
  Constant1 : Constant  Value=2  OutDataTypeStr=Inherit: Inherit via back propagation  SampleTime=-1
  Constant2 : Constant  Value=2  OutDataTypeStr=Inherit: Inherit via back propagation  SampleTime=-1
  Delay{,1..12} (13 alike) : Delay  DelayLength=1
  Logical Operator : Logic  Operator=OR  AllPortsSameDT=off  OutDataTypeStr=boolean
  Switch : Switch  Criteria=u2 ~= 0
  Switch1 : Switch  Criteria=u2 ~= 0
  A2 : Outport
  index : Outport  Port=2
  wires:
  Compare To Constant/1 -> Delay2/1
  Compare To Constant1/1 -> Delay3/1
  Logical Operator/1 -> Delay6/1
  A1/1 -> Delay1/1
  Switch/1 -> A2/1
  Constant/1 -> Add/2
  Add/1 -> Delay8/1
  Add2/1 -> Delay11/1
  Constant1/1 -> Add2/2
  Switch1/1 -> index/1
  Constant2/1 -> Add3/2
  Index/1 -> Delay/1
  Add3/1 -> Delay12/1
  Delay/1 -> Compare To Constant/1, Compare To Constant1/1, Delay9/1, Delay10/1
  Delay1/1 -> Delay5/1, Delay4/1
  Delay2/1 -> Logical Operator/1
  Delay3/1 -> Logical Operator/2
  Delay4/1 -> Delay7/1
  Delay5/1 -> Add/1
  Delay6/1 -> Switch1/2, Switch/2
  Delay7/1 -> Switch/1
  Delay8/1 -> Switch/3
  Delay9/1 -> Add2/1
  Delay10/1 -> Add3/1
  Delay11/1 -> Switch1/1
  Delay12/1 -> Switch1/3

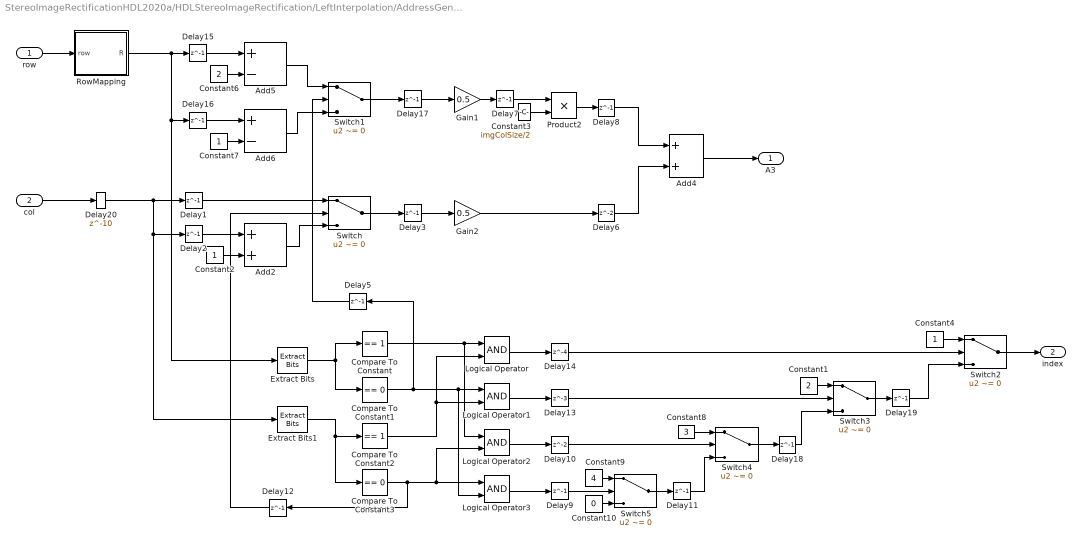
== system StereoImageRectificationHDL2020a/HDLStereoImageRectification/LeftInterpolation/AddressGeneration/AddressCalculation/Pix3Add ==
  row : Inport
  col : Inport  Port=2
  Add2 : Sum  OutDataTypeStr=Inherit: Same as first input
  Add4 : Sum  OutDataTypeStr=Inherit: Same as first input
  Add5 : Sum  Inputs=+-  OutDataTypeStr=Inherit: Same as first input
  Add6 : Sum  Inputs=+-  OutDataTypeStr=Inherit: Same as first input
  Compare To Constant : simulink/Logic and Bit Operations/Compare To Constant  relop===  const=1  OutDataTypeStr=boolean
  Compare To Constant1 : simulink/Logic and Bit Operations/Compare To Constant  relop===  const=0  OutDataTypeStr=boolean
  Compare To Constant2 : simulink/Logic and Bit Operations/Compare To Constant  relop===  const=1  OutDataTypeStr=boolean
  Compare To Constant3 : simulink/Logic and Bit Operations/Compare To Constant  relop===  const=0  OutDataTypeStr=boolean
  Constant1 : Constant  Value=2  OutDataTypeStr=uint8  SampleTime=-1
  Constant10 : Constant  Value=0  OutDataTypeStr=uint8  SampleTime=-1
  Constant2 : Constant  OutDataTypeStr=Inherit: Inherit via back propagation  SampleTime=-1
  Constant3 : Constant  Value=imgColSize/2  OutDataTypeStr=uint32  SampleTime=-1
  Constant4 : Constant  OutDataTypeStr=uint8  SampleTime=-1
  Constant6 : Constant  Value=2  OutDataTypeStr=Inherit: Inherit via back propagation  SampleTime=-1
  Constant7 : Constant  OutDataTypeStr=Inherit: Inherit via back propagation  SampleTime=-1
  Constant8 : Constant  Value=3  OutDataTypeStr=uint8  SampleTime=-1
  Constant9 : Constant  Value=4  OutDataTypeStr=uint8  SampleTime=-1
  Delay{1..3,5,7..9,11..12,15..19} (14 alike) : Delay  DelayLength=1
  Delay10 : Delay
  Delay13 : Delay  DelayLength=3
  Delay14 : Delay  DelayLength=4
  Delay20 : Delay  DelayLength=10
  Delay6 : Delay
  Extract Bits : simulink/Logic and Bit Operations/Extract Bits  bitsToExtract=Range ending with least significant bit  numBits=1  bitIdxRange=[0 7]  outScalingMode=Preserve fixed-point scaling
  Extract Bits1 : simulink/Logic and Bit Operations/Extract Bits  bitsToExtract=Range ending with least significant bit  numBits=1  bitIdxRange=[0 7]  outScalingMode=Preserve fixed-point scaling
  Gain1 : Gain  Gain=0.5  OutDataTypeStr=Inherit: Inherit via back propagation
  Gain2 : Gain  Gain=0.5  OutDataTypeStr=Inherit: Inherit via back propagation
  Logical Operator{,1..3} (4 alike) : Logic  AllPortsSameDT=off  OutDataTypeStr=boolean
  Product2 : Product  OutDataTypeStr=Inherit: Inherit via back propagation
  RowMapping : Subsystem
  Switch{,1..5} (6 alike) : Switch  Criteria=u2 ~= 0
  A3 : Outport
  index : Outport  Port=2
  wires:
  Gain2/1 -> Delay6/1
  Switch/1 -> Delay3/1
  Delay3/1 -> Gain2/1
  Delay2/1 -> Add2/1
  Constant2/1 -> Add2/2
  Delay1/1 -> Switch/1
  Add2/1 -> Switch/3
  Delay5/1 -> Switch1/2
  Delay17/1 -> Gain1/1
  Switch1/1 -> Delay17/1
  Add6/1 -> Switch1/3
  Add5/1 -> Switch1/1
  Constant7/1 -> Add6/2
  Delay16/1 -> Add6/1
  Delay15/1 -> Add5/1
  Constant6/1 -> Add5/2
  Gain1/1 -> Delay7/1
  Constant3/1 -> Product2/2
  Delay7/1 -> Product2/1
  Product2/1 -> Delay8/1
  Delay8/1 -> Add4/1
  Delay6/1 -> Add4/2
  Add4/1 -> A3/1
  Extract Bits/1 -> Compare To Constant/1, Compare To Constant1/1
  Extract Bits1/1 -> Compare To Constant3/1, Compare To Constant2/1
  Compare To Constant/1 -> Logical Operator2/1, Logical Operator/1
  Compare To Constant2/1 -> Logical Operator1/2, Logical Operator/2
  Compare To Constant1/1 -> Delay5/1, Logical Operator3/2, Logical Operator1/1
  Switch2/1 -> index/1
  Compare To Constant3/1 -> Logical Operator3/1, Logical Operator2/2, Delay12/1
  Delay12/1 -> Switch/2
  col/1 -> Delay20/1
  Delay14/1 -> Switch2/2
  Delay11/1 -> Switch4/3
  Delay19/1 -> Switch2/3
  Switch5/1 -> Delay11/1
  Delay9/1 -> Switch5/2
  Constant1/1 -> Switch3/1
  Constant10/1 -> Switch5/3
  Delay13/1 -> Switch3/2
  Constant4/1 -> Switch2/1
  Switch4/1 -> Delay18/1
  Delay10/1 -> Switch4/2
  Constant9/1 -> Switch5/1
  Switch3/1 -> Delay19/1
  Constant8/1 -> Switch4/1
  Delay18/1 -> Switch3/3
  Logical Operator3/1 -> Delay9/1
  Logical Operator2/1 -> Delay10/1
  Logical Operator1/1 -> Delay13/1
  Logical Operator/1 -> Delay14/1
  RowMapping/1(R) -> Delay15/1, Extract Bits/1, Delay16/1
  row/1 -> RowMapping/1(row)
  Delay20/1 -> Delay1/1, Extract Bits1/1, Delay2/1

== system StereoImageRectificationHDL2020a/HDLStereoImageRectification/LeftInterpolation/AddressGeneration/AddressCalculation/Pix4Add ==
  A3 : Inport
  Index : Inport  Port=2
  Add : Sum  OutDataTypeStr=Inherit: Inherit via back propagation
  Add2 : Sum  OutDataTypeStr=Inherit: Inherit via back propagation
  Add3 : Sum  Inputs=+-  OutDataTypeStr=Inherit: Inherit via back propagation
  Compare To Constant : simulink/Logic and Bit Operations/Compare To Constant  relop===  const=1  OutDataTypeStr=boolean
  Compare To Constant1 : simulink/Logic and Bit Operations/Compare To Constant  relop===  const=2  OutDataTypeStr=boolean
  Constant : Constant  OutDataTypeStr=Inherit: Inherit via back propagation  SampleTime=-1
  Constant1 : Constant  Value=2  OutDataTypeStr=Inherit: Inherit via back propagation  SampleTime=-1
  Constant2 : Constant  Value=2  OutDataTypeStr=Inherit: Inherit via back propagation  SampleTime=-1
  Delay{,1..12} (13 alike) : Delay  DelayLength=1
  Logical Operator : Logic  Operator=OR  AllPortsSameDT=off  OutDataTypeStr=boolean
  Switch : Switch  Criteria=u2 ~= 0
  Switch1 : Switch  Criteria=u2 ~= 0
  A4 : Outport
  index : Outport  Port=2
  wires:
  Compare To Constant/1 -> Delay2/1
  Compare To Constant1/1 -> Delay3/1
  Logical Operator/1 -> Delay6/1
  A3/1 -> Delay1/1
  Switch/1 -> A4/1
  Constant/1 -> Add/2
  Add/1 -> Delay8/1
  Add2/1 -> Delay11/1
  Constant1/1 -> Add2/2
  Switch1/1 -> index/1
  Constant2/1 -> Add3/2
  Index/1 -> Delay/1
  Add3/1 -> Delay12/1
  Delay/1 -> Compare To Constant/1, Compare To Constant1/1, Delay9/1, Delay10/1
  Delay1/1 -> Delay5/1, Delay4/1
  Delay2/1 -> Logical Operator/1
  Delay3/1 -> Logical Operator/2
  Delay4/1 -> Delay7/1
  Delay5/1 -> Add/1
  Delay6/1 -> Switch1/2, Switch/2
  Delay7/1 -> Switch/1
  Delay8/1 -> Switch/3
  Delay9/1 -> Add2/1
  Delay10/1 -> Add3/1
  Delay11/1 -> Switch1/1
  Delay12/1 -> Switch1/3

== system StereoImageRectificationHDL2020a/HDLStereoImageRectification/RightInterpolation/AddressGeneration/AddressCalculation/CappingAddress ==
  row : Inport
  col : Inport  Port=2
  AND1 : Logic  IconShape=distinctive  AllPortsSameDT=off  OutDataTypeStr=boolean
  AND2 : Logic  IconShape=distinctive  AllPortsSameDT=off  OutDataTypeStr=boolean
  Compare To Constant3 : simulink/Logic and Bit Operations/Compare To Constant  relop=<=  const=1  OutDataTypeStr=boolean
  Compare To Constant4 : simulink/Logic and Bit Operations/Compare To Constant  relop=<=  const=dimOut(2)-1  OutDataTypeStr=boolean
  Compare To Constant5 : simulink/Logic and Bit Operations/Compare To Constant  relop=>  const=1  OutDataTypeStr=boolean
  Compare To Constant6 : simulink/Logic and Bit Operations/Compare To Constant  relop=<=  const=1  OutDataTypeStr=boolean
  Compare To Constant7 : simulink/Logic and Bit Operations/Compare To Constant  relop=<=  const=dimOut(1)-1  OutDataTypeStr=boolean
  Compare To Constant8 : simulink/Logic and Bit Operations/Compare To Constant  relop=>  const=1  OutDataTypeStr=boolean
  Constant1 : Constant  Value=dimOut(2)-1  OutDataTypeStr=Inherit: Inherit via back propagation  SampleTime=-1
  Constant2 : Constant  Value=dimOut(1)-1  OutDataTypeStr=Inherit: Inherit via back propagation  SampleTime=-1
  Constant3 : Constant  OutDataTypeStr=Inherit: Inherit via back propagation  SampleTime=-1
  Constant4 : Constant  OutDataTypeStr=Inherit: Inherit via back propagation  SampleTime=-1
  Delay{,1..17} (18 alike) : Delay  DelayLength=1
  Switch{2..5} (4 alike) : Switch  Criteria=u2 ~= 0  OutDataTypeStr=Inherit: Inherit via back propagation
  r : Outport
  c : Outport  Port=2
  wires:
  col/1 -> Compare To Constant5/1, Compare To Constant4/1, Delay3/1, Delay6/1
  Compare To Constant5/1 -> Delay1/1
  Switch2/1 -> Delay5/1
  Constant3/1 -> Switch3/1
  Compare To Constant4/1 -> Delay/1
  AND1/1 -> Delay2/1
  Constant1/1 -> Switch2/3
  Compare To Constant3/1 -> Delay8/1
  Delay/1 -> AND1/1
  Delay1/1 -> AND1/2
  Delay2/1 -> Switch2/2
  Delay3/1 -> Delay4/1
  Delay4/1 -> Switch2/1
  Delay5/1 -> Switch3/3
  Delay6/1 -> Delay7/1
  Delay7/1 -> Compare To Constant3/1
  Delay8/1 -> Switch3/2
  Delay17/1 -> Switch5/2
  Delay10/1 -> AND2/2
  Delay14/1 -> Switch5/3
  Delay15/1 -> Delay16/1
  Delay12/1 -> Delay13/1
  Delay13/1 -> Switch4/1
  Delay11/1 -> Switch4/2
  Delay16/1 -> Compare To Constant6/1
  Switch4/1 -> Delay14/1
  row/1 -> Delay15/1, Compare To Constant8/1, Compare To Constant7/1, Delay12/1
  Compare To Constant8/1 -> Delay10/1
  Constant2/1 -> Switch4/3
  AND2/1 -> Delay11/1
  Compare To Constant6/1 -> Delay17/1
  Constant4/1 -> Switch5/1
  Compare To Constant7/1 -> Delay9/1
  Delay9/1 -> AND2/1
  Switch3/1 -> c/1
  Switch5/1 -> r/1

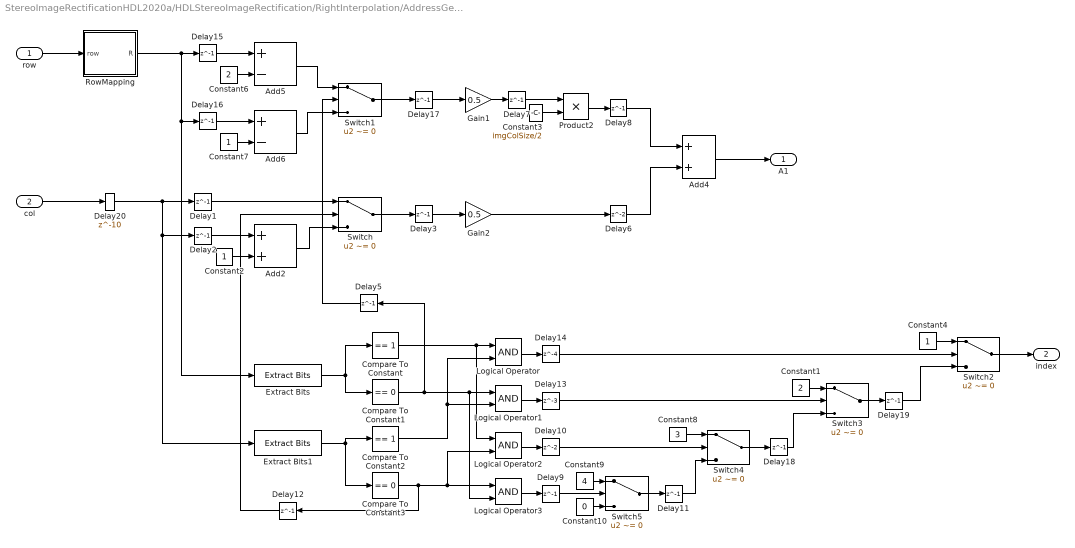
== system StereoImageRectificationHDL2020a/HDLStereoImageRectification/RightInterpolation/AddressGeneration/AddressCalculation/Pix1Add ==
  row : Inport
  col : Inport  Port=2
  Add2 : Sum  OutDataTypeStr=Inherit: Same as first input
  Add4 : Sum  OutDataTypeStr=Inherit: Same as first input
  Add5 : Sum  Inputs=+-  OutDataTypeStr=Inherit: Same as first input
  Add6 : Sum  Inputs=+-  OutDataTypeStr=Inherit: Same as first input
  Compare To Constant : simulink/Logic and Bit Operations/Compare To Constant  relop===  const=1  OutDataTypeStr=boolean
  Compare To Constant1 : simulink/Logic and Bit Operations/Compare To Constant  relop===  const=0  OutDataTypeStr=boolean
  Compare To Constant2 : simulink/Logic and Bit Operations/Compare To Constant  relop===  const=1  OutDataTypeStr=boolean
  Compare To Constant3 : simulink/Logic and Bit Operations/Compare To Constant  relop===  const=0  OutDataTypeStr=boolean
  Constant1 : Constant  Value=2  OutDataTypeStr=uint8  SampleTime=-1
  Constant10 : Constant  Value=0  OutDataTypeStr=uint8  SampleTime=-1
  Constant2 : Constant  OutDataTypeStr=Inherit: Inherit via back propagation  SampleTime=-1
  Constant3 : Constant  Value=imgColSize/2  OutDataTypeStr=uint32  SampleTime=-1
  Constant4 : Constant  OutDataTypeStr=uint8  SampleTime=-1
  Constant6 : Constant  Value=2  OutDataTypeStr=Inherit: Inherit via back propagation  SampleTime=-1
  Constant7 : Constant  OutDataTypeStr=Inherit: Inherit via back propagation  SampleTime=-1
  Constant8 : Constant  Value=3  OutDataTypeStr=uint8  SampleTime=-1
  Constant9 : Constant  Value=4  OutDataTypeStr=uint8  SampleTime=-1
  Delay{1..3,5,7..9,11..12,15..19} (14 alike) : Delay  DelayLength=1
  Delay10 : Delay
  Delay13 : Delay  DelayLength=3
  Delay14 : Delay  DelayLength=4
  Delay20 : Delay  DelayLength=10
  Delay6 : Delay
  Extract Bits : simulink/Logic and Bit Operations/Extract Bits  bitsToExtract=Range ending with least significant bit  numBits=1  bitIdxRange=[0 7]  outScalingMode=Preserve fixed-point scaling
  Extract Bits1 : simulink/Logic and Bit Operations/Extract Bits  bitsToExtract=Range ending with least significant bit  numBits=1  bitIdxRange=[0 7]  outScalingMode=Preserve fixed-point scaling
  Gain1 : Gain  Gain=0.5  OutDataTypeStr=Inherit: Inherit via back propagation
  Gain2 : Gain  Gain=0.5  OutDataTypeStr=Inherit: Inherit via back propagation
  Logical Operator{,1..3} (4 alike) : Logic  AllPortsSameDT=off  OutDataTypeStr=boolean
  Product2 : Product  OutDataTypeStr=Inherit: Inherit via back propagation
  RowMapping : Subsystem
  Switch{,1..5} (6 alike) : Switch  Criteria=u2 ~= 0
  A1 : Outport
  index : Outport  Port=2
  wires:
  col/1 -> Delay20/1
  Delay12/1 -> Switch/2
  Compare To Constant3/1 -> Delay12/1, Logical Operator2/2, Logical Operator3/1
  Switch2/1 -> index/1
  Logical Operator3/1 -> Delay9/1
  Logical Operator2/1 -> Delay10/1
  Logical Operator1/1 -> Delay13/1
  Logical Operator/1 -> Delay14/1
  Compare To Constant1/1 -> Logical Operator1/1, Logical Operator3/2, Delay5/1
  Compare To Constant2/1 -> Logical Operator/2, Logical Operator1/2
  Compare To Constant/1 -> Logical Operator/1, Logical Operator2/1
  Extract Bits1/1 -> Compare To Constant3/1, Compare To Constant2/1
  Extract Bits/1 -> Compare To Constant/1, Compare To Constant1/1
  Add4/1 -> A1/1
  Delay6/1 -> Add4/2
  Delay8/1 -> Add4/1
  Product2/1 -> Delay8/1
  Delay7/1 -> Product2/1
  Constant3/1 -> Product2/2
  Gain1/1 -> Delay7/1
  Constant6/1 -> Add5/2
  Delay15/1 -> Add5/1
  Delay16/1 -> Add6/1
  Constant7/1 -> Add6/2
  row/1 -> RowMapping/1(row)
  Add5/1 -> Switch1/1
  Add6/1 -> Switch1/3
  Switch1/1 -> Delay17/1
  Delay17/1 -> Gain1/1
  Delay5/1 -> Switch1/2
  Add2/1 -> Switch/3
  Delay1/1 -> Switch/1
  Constant2/1 -> Add2/2
  Delay2/1 -> Add2/1
  Delay3/1 -> Gain2/1
  Switch/1 -> Delay3/1
  Gain2/1 -> Delay6/1
  Constant1/1 -> Switch3/1
  Constant4/1 -> Switch2/1
  Switch3/1 -> Delay19/1
  Switch4/1 -> Delay18/1
  Constant8/1 -> Switch4/1
  Constant9/1 -> Switch5/1
  Switch5/1 -> Delay11/1
  Constant10/1 -> Switch5/3
  Delay9/1 -> Switch5/2
  Delay10/1 -> Switch4/2
  Delay13/1 -> Switch3/2
  Delay14/1 -> Switch2/2
  Delay11/1 -> Switch4/3
  Delay18/1 -> Switch3/3
  Delay19/1 -> Switch2/3
  RowMapping/1(R) -> Extract Bits/1, Delay16/1, Delay15/1
  Delay20/1 -> Extract Bits1/1, Delay2/1, Delay1/1

== system StereoImageRectificationHDL2020a/HDLStereoImageRectification/RightInterpolation/AddressGeneration/AddressCalculation/Pix2Add ==
  A1 : Inport
  Index : Inport  Port=2
  Add : Sum  OutDataTypeStr=Inherit: Inherit via back propagation
  Add2 : Sum  OutDataTypeStr=Inherit: Inherit via back propagation
  Add3 : Sum  Inputs=+-  OutDataTypeStr=Inherit: Inherit via back propagation
  Compare To Constant : simulink/Logic and Bit Operations/Compare To Constant  relop===  const=1  OutDataTypeStr=boolean
  Compare To Constant1 : simulink/Logic and Bit Operations/Compare To Constant  relop===  const=2  OutDataTypeStr=boolean
  Constant : Constant  OutDataTypeStr=Inherit: Inherit via back propagation  SampleTime=-1
  Constant1 : Constant  Value=2  OutDataTypeStr=Inherit: Inherit via back propagation  SampleTime=-1
  Constant2 : Constant  Value=2  OutDataTypeStr=Inherit: Inherit via back propagation  SampleTime=-1
  Delay{,1..12} (13 alike) : Delay  DelayLength=1
  Logical Operator : Logic  Operator=OR  AllPortsSameDT=off  OutDataTypeStr=boolean
  Switch : Switch  Criteria=u2 ~= 0
  Switch1 : Switch  Criteria=u2 ~= 0
  A2 : Outport
  index : Outport  Port=2
  wires:
  Compare To Constant/1 -> Delay2/1
  Compare To Constant1/1 -> Delay3/1
  Logical Operator/1 -> Delay6/1
  A1/1 -> Delay1/1
  Switch/1 -> A2/1
  Constant/1 -> Add/2
  Add/1 -> Delay8/1
  Add2/1 -> Delay11/1
  Constant1/1 -> Add2/2
  Switch1/1 -> index/1
  Constant2/1 -> Add3/2
  Index/1 -> Delay/1
  Add3/1 -> Delay12/1
  Delay/1 -> Compare To Constant/1, Compare To Constant1/1, Delay9/1, Delay10/1
  Delay1/1 -> Delay5/1, Delay4/1
  Delay2/1 -> Logical Operator/1
  Delay3/1 -> Logical Operator/2
  Delay4/1 -> Delay7/1
  Delay5/1 -> Add/1
  Delay6/1 -> Switch1/2, Switch/2
  Delay7/1 -> Switch/1
  Delay8/1 -> Switch/3
  Delay9/1 -> Add2/1
  Delay10/1 -> Add3/1
  Delay11/1 -> Switch1/1
  Delay12/1 -> Switch1/3
